simulink model "mj_monitorTune_ROS"  (R2025a)
settings: Solver=FixedStepDiscrete  StartTime=0.0  StopTime=inf  RelTol=1e-3
model workspace (MAT data in the model file):
  SL_ROS_VariableLengthArrays_MaxSizes.CommonInfo.ArrayTruncateAction = 'EmitWarning'
  SL_ROS_VariableLengthArrays_MaxSizes.MsgTypeMap = containers.Map
  SL_ROS_VariableLengthArrays_MaxSizes.MsgTypeMap.serialization.keys = {'sensor_msgs/Image'}
  SL_ROS_VariableLengthArrays_MaxSizes.MsgTypeMap.serialization.values{1}(1).PropertyName = 'data'
  SL_ROS_VariableLengthArrays_MaxSizes.MsgTypeMap.serialization.values{1}(1).DataType = 'uint8'
  SL_ROS_VariableLengthArrays_MaxSizes.MsgTypeMap.serialization.values{1}(1).MaxLength = 940000
  SL_ROS_VariableLengthArrays_MaxSizes.MsgTypeMap.serialization.values{1}(2).PropertyName = 'encoding'
  SL_ROS_VariableLengthArrays_MaxSizes.MsgTypeMap.serialization.values{1}(2).DataType = 'uint8'
  SL_ROS_VariableLengthArrays_MaxSizes.MsgTypeMap.serialization.values{1}(2).MaxLength = 128
  SL_ROS_VariableLengthArrays_MaxSizes.MsgTypeMap.serialization.uniformity = 0
  SL_ROS_VariableLengthArrays_MaxSizes.MsgTypeMap.serialization.keyType = 'char'
  SL_ROS_VariableLengthArrays_MaxSizes.MsgTypeMap.serialization.valueType = 'any'
undefined symbols (not defined in the file or in its folder): coder, orientation, ros
libraries: ros2lib x5, mjLib x2
settings Model: SimulationMode=external  Creator=MuJoCo Simulink Blockset  LastModifiedBy=turbo
settings SolverCC: MinimalZcImpactIntegration=on
settings DataIOCC: DSMLogging=off
settings OptimizationCC: EnhancedBackFolding=on  PassReuseOutputArgsThreshold=0.0  ZeroExternalMemoryAtStartup=off  ZeroInternalMemoryAtStartup=off  MaxStackSize=64  OptimizeBlockOrder=speed  DifferentSizesBufferReuse=on  OptimizationCustomize=off
settings DebuggingCC: ReadBeforeWriteMsg=DisableAll  WriteAfterWriteMsg=DisableAll  WriteAfterReadMsg=DisableAll  MultiTaskDSMMsg=none  ParameterTunabilityLossMsg=error
settings HardwareCC: ProdBitPerLong=64.0  ProdLargestAtomicInteger=LongLong  ProdLargestAtomicFloat=Double  ProdLongLongMode=on  ProdHWDeviceType=ARM Compatible->ARM Cortex-A (64-bit)  TargetBitPerLong=64.0  TargetBitPerPointer=64.0  TargetBitPerSizeT=64.0  TargetBitPerPtrDiffT=64.0  TargetLargestAtomicInteger=LongLong  TargetLargestAtomicFloat=Double  TargetLongLongMode=on  TargetIntDivRoundTo=Zero  TargetEndianess=LittleEndian  TargetWordSize=64.0  TargetHWDeviceType=ARM Compatible->ARM Cortex-A (64-bit)  ProdEqTarget=off
settings ModelReferenceCC: UpdateModelReferenceTargets=IfOutOfDate  EnableRefExpFcnMdlSchedulingChecks=on
settings SFSimCC: SFSimEcho=off  MATLABDynamicMemAlloc=off  SimTargetLang=C++  SimDLTargetLibrary=mkl-dnn
settings RTWCC: SystemTargetFile=ert.tlc  HardwareBoard=Robot Operating System 2 (ROS 2)  TLCOptions="-aInlineSetEventsForThisBaseRateFcn=TLC_FALSE -aSuppressMultiTaskScheduler=TLC_FALSE  -aRateBasedStepFcn=0"  TemplateMakefile=ert_default_tmf  PostCodeGenCommand=mj_postcodegen(buildInfo);codertarget.postCodeGenHookCommand(h)  GenerateReport=on  Toolchain=Colcon Tools  BuildConfiguration=Faster Runs  LaunchReport=on  TargetLang=C++  GPUComputeCapability=3.5  DLArmComputeVersion=19.05  Description=Embedded Coder
settings CodeAppCC: ForceParamTrailComments=on  OperatorAnnotations=on
settings ERTTargetCC: ExtModeTransport=0.0  ExtModeStaticAlloc=off  ExtModeMexFile=ext_comm  ExtModeIntrfLevel=Level1  InlinedParameterPlacement=Hierarchical  RootIOFormat=Structure reference  DynamicArrayContainerType=coder::array  ERTCustomFileBanners=off  SupportContinuousTime=on  SupportNonInlinedSFcns=on  RemoveResetFunc=off  ModelStepFunctionPrototypeControlCompliant=off

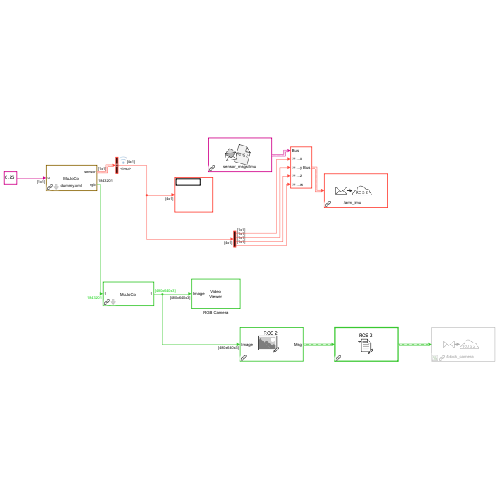
[thumbnail: Simulink's stored preview of the top-level diagram]
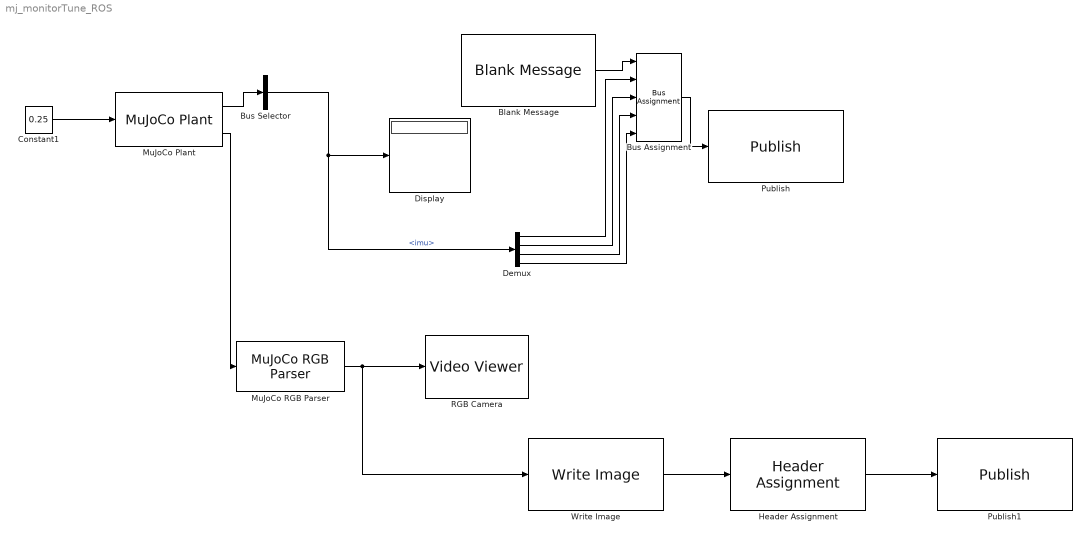
== system mj_monitorTune_ROS ==
  Blank Message : ros2lib/Blank Message  messageClass=Message  entityType=sensor_msgs/Imu  messageType=sensor_msgs/Imu  SampleTime=inf
  Bus Assignment : BusAssignment  AssignedSignals=orientation.x,orientation.y,orientation.z,orientation.w
  Bus Selector : BusSelector  OutputSignals=imu
  Constant1 : Constant  Value=0.25
  Demux : Demux
  Display : Display
  Header Assignment : ros2lib/Header Assignment  SetFrameID=on  FrameID=block_frame  InsertTimeStamp=on  SetHeaderFieldName=Use the default header field name  HeaderFieldName=header
  MuJoCo Plant : mjLib/MuJoCo Plant  VariantControl=rgbOutOption  controlBus=[]  sensorBus=[]  controlLength=[]  sensorLength=[]  rgbLength=[]  depthLength=[]  segLength=[]  sampleTime=0.005  xmlFileRel=dummy.xml  xmlFile=dummy.xml  renderingType=Local  vsync=off  visualFPS=60  zoomLevel=1  keyframeName='home'  znear=0.059256  zfar=296.2816  cameraSampleTime=0.20  rgbOutOption=on  depthOutOption=off  segmentationOutOption=off  controlInterfaceType=Vector
      settings: SourceProductName=MuJoCo Simulator
  MuJoCo RGB Parser : mjLib/MuJoCo RGB Parser  inputBusType=mj_bus_rgb_3624495926710663437  selectedCamera=camera  imageRows=480  imageCols=640  startingIndex=921601  endingIndex=1843200
      settings: SourceProductName=MuJoCo Simulator
  Publish : ros2lib/Publish  topicSource=Specify your own  topic=/arm_imu  messageType=sensor_msgs/Imu  QOSHistory=Keep last  QOSDepth=2  QOSReliability=Reliable  QOSDurability=Volatile  QOSDeadline=Inf  QOSLifespan=Inf  QOSLiveliness=Automatic  QOSLeaseDuration=Inf  QOSAvoidROSNamespaceConventions=off
  Publish1 : ros2lib/Publish  topicSource=Specify your own  topic=/block_camera  messageType=sensor_msgs/Image  QOSHistory=Keep last  QOSDepth=1  QOSReliability=Reliable  QOSDurability=Volatile  QOSDeadline=Inf  QOSLifespan=Inf  QOSLiveliness=Automatic  QOSLeaseDuration=Inf  QOSAvoidROSNamespaceConventions=off
  RGB Camera : VideoViewer  FigPos=[1403 782 418 304]
  Write Image : ros2lib/Write Image  ImageEncoding=rgb8  EncodingStruct=ros.msg.sensor_msgs.internal.ImageEncoding.info(coder.const('rgb8'))  HasAlpha=off  messageType=sensor_msgs/Image
  wires:
  Constant1/1 -> MuJoCo Plant/1
  MuJoCo Plant/1 -> Bus Selector/1
  Bus Selector/1 -> Demux/1, Display/1  "<imu>"
  Bus Assignment/1 -> Publish/1
  Blank Message/1 -> Bus Assignment/1
  Demux/4 -> Bus Assignment/5
  Demux/3 -> Bus Assignment/4
  Demux/2 -> Bus Assignment/3
  Demux/1 -> Bus Assignment/2
  MuJoCo RGB Parser/1 -> Write Image/1, RGB Camera/1
  MuJoCo Plant/2 -> MuJoCo RGB Parser/1
  Write Image/1 -> Header Assignment/1
  Header Assignment/1 -> Publish1/1
